simulink model "Antenna_Simulink_Block"  (R2019b)
settings: Solver=VariableStepAuto  StartTime=0.0  StopTime=0  RelTol=1e-3
undefined symbols (not defined in the file or in its folder): physconst
libraries: rfBudgetAnalyzer_lib x5, simrfV2elements x3, simrfV2util1 x3, simrfV2sources1 x1
settings Model: Creator=BLAUZON3  LastModifiedBy=BLAUZON3

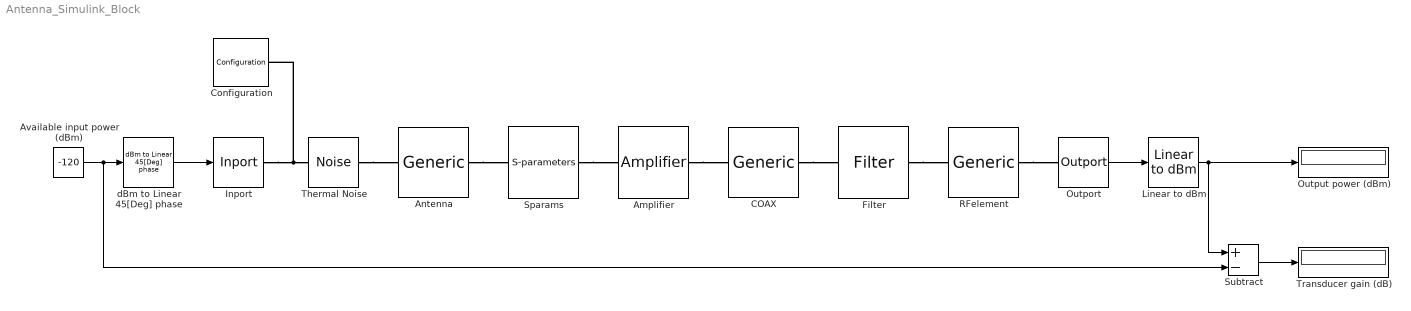
== system Antenna_Simulink_Block ==
  Amplifier : simrfV2elements/Amplifier  classname=amplifier  DataSource=Data file  File=unitygain.s2p  Paramtype=S-parameters  Sparam=[0 0;1 0]  SparamFreq=1e9 Hz  SparamZ0=50  Residues=0  Poles=0  DF={0 0; 1 0}  Source_linear_gain=Available power gain  linear_gain=12 dB  Zin=50  Zout=50  Source_Poly=Even and odd order  Poly_Coeffs=[0 1]  IPType=Output  IP2=Inf dBm  IP3=Inf dBm  P1dB=inf dBm  Psat=inf dBm  Gcomp=inf dBm  InternalGrounding=on  SourceFreq=Extracted from data source  PlotFreq=[1e9:1e6:3e9] Hz  PlotType=X-Y plane  YParam1=S11  YFormat1=Magnitude (decibels)  YParam2=None  YFormat2=Magnitude (decibels)  YOption=Linear  XOption=Linear  SparamRepresentation=Time domain (rationalfit)  FitTol=-40  FitOpt=Fit individually  AutoImpulseLength=on  ImpulseLength=1e-10 s  MagModeling=off  AddNoise=on  NoiseType=Noise figure  NoiseDist=White  NF=0  MinNF=0  Gopt=0  RN=0  CarrierFreq=0 Hz  NoiseAutoImpulseLength=on  NoiseImpulseLength=1e-10 s  SpecifyOpFreq=off  OpFreq=0 Hz
      settings: SourceProductName=RF Blockset  SourceProductBaseCode=RB
  Antenna : rfBudgetAnalyzer_lib/Generic  Gain=24  NF=0  OIP3=Inf  Zin=50  Zout=50
      settings: SourceProductName=RF Blockset  SourceProductBaseCode=RB
  Available input power (dBm) : Constant  Value=-120
  COAX : rfBudgetAnalyzer_lib/Generic  Gain=-6  NF=0  OIP3=Inf  Zin=50  Zout=50
      settings: SourceProductName=RF Blockset  SourceProductBaseCode=RB
  Configuration : simrfV2util1/Configuration  AutoFreq=on  Tones=[] Hz  Harmonics=[]  NormalizeCarrierPower=on  SolverType=Auto  UseCCode=on  StepSize=(1/20000000)/8 s  AddNoise=on  defaultRNG=on  Seed=0  Temperature=290.0 K  SolverDelFlag=0  AbsTol=1e-6  RelTol=1e-3  MaxIter=10  ErrorEstimationType=2-norm over all variables  EnableInterpFilter=on  HiddenFIRfilterControllerParam=off  SmallSignalApprox=off  AllSimFreqs=on  SimFreqs=[] Hz  SimFreqsInternal=[]  SamplesPerFrame=1
      settings: SourceProductName=RF Blockset  SourceProductBaseCode=RB
  Filter : simrfV2elements/Filter  classname=filter  DesignMethod=Butterworth  ResponseType=Bandpass  Implementation=LC Tee  ImplementationIdeal=Constant per carrier  ImplementationRational=Transfer function  UseFilterOrder=on  FilterOrder=3  PassFreq_lp=1 GHz  PassFreq_hp=2 GHz  PassFreq_bp=[5.8 6] GHz  PassFreq_bs=[1 4] GHz  PassAtten=3.0103  StopFreq_lp=2 GHz  StopFreq_hp=1 GHz  StopFreq_bp=[1.5 3.5] GHz  StopFreq_bs=[2.1 2.9] GHz  StopAtten=40  Rsrc=50  Rload=50  AutoImpulseLength=on  ImpulseLength=1e-10 s  InternalGrounding=on  PlotFuncLeft=Voltage transfer  PlotLeftForm=Magnitude (decibels)  PlotRightOnVT=None  PlotRightNoTD=None  PlotRightNoGD=None  PlotRightNoIR=None  PlotRightNoSR=None  PlotRightForm=Magnitude (decibels)  FreqPoints=logspace(0,10,101)  Freq_unit=Hz  TimePoints=linspace(0,1,1e6+1)  Time_unit=s  XaxisScale=Linear  YaxisScale=Linear
      settings: SourceProductName=RF Blockset  SourceProductBaseCode=RB
  Inport : simrfV2util1/Inport  SimulinkInputSignalType=Power  CarrierFreq=5.9 GHz  ZS=50  InternalGrounding=on
      settings: SourceProductName=RF Blockset  SourceProductBaseCode=RB
  Linear to dBm : rfBudgetAnalyzer_lib/Linear to dBm  SystemSampleTime=-1  Latency=0  AutoFrameSizeCalculation=off
      settings: SourceProductName=RF Blockset  SourceProductBaseCode=RB
  Outport : simrfV2util1/Outport  SensorType=Power  OutputFormat=Complex Baseband  CarrierFreq=5.9 GHz  ZL=50  InternalGrounding=on  StepSize=1e-6 s  AutoStep=on
      settings: SourceProductName=RF Blockset  SourceProductBaseCode=RB
  Output power (dBm) : Display
  RFelement : rfBudgetAnalyzer_lib/Generic  Gain=0  NF=0  OIP3=Inf  Zin=50  Zout=50
      settings: SourceProductName=RF Blockset  SourceProductBaseCode=RB
  Sparams : simrfV2elements/S-parameters  classname=sparam_element  DataSource=Data file  File=sparam.s2p  Paramtype=S-parameters  Sparam=[0 0;1 0]  SparamFreq=1e9 Hz  SparamZ0=50  Residues=0  Poles=0  DF={0 0; 1 0}  FitOpt=Share all poles  FitTol=-40  SourceFreq=Extracted from data source  PlotFreq=[1e9:1e6:3e9] Hz  PlotType=X-Y plane  YParam1=S11  YFormat1=Magnitude (decibels)  YParam2=None  YFormat2=Magnitude (decibels)  YOption=Linear  XOption=Linear  AddNoise=on  InternalGrounding=on  SparamRepresentation=Time domain (rationalfit)  AutoImpulseLength=on  ImpulseLength=1e-10 s  MagModeling=off
      settings: SourceProductName=RF Blockset  SourceProductBaseCode=RB
  Subtract : Sum  Inputs=+-
  Thermal Noise : simrfV2sources1/Noise  SimulinkInputSignalType=Ideal voltage  NoiseType=White  NoisePSD=4*physconst('Boltzmann')*290*50  CarrierFreq=0 Hz  AutoImpulseLength=on  ImpulseLength=1e-10 s  InternalGrounding=off
      settings: SourceProductName=RF Blockset  SourceProductBaseCode=RB
  Transducer gain (dB) : Display
  dBm to Linear 45[Deg] phase : rfBudgetAnalyzer_lib/dBm to Linear 45[Deg] phase  SystemSampleTime=-1  Latency=0  AutoFrameSizeCalculation=off
      settings: SourceProductName=RF Blockset  SourceProductBaseCode=RB
  wires:
  Available input power (dBm)/1 -> dBm to Linear 45[Deg] phase/1, Subtract/2
  dBm to Linear 45[Deg] phase/1 -> Inport/1
  Outport/1 -> Linear to dBm/1
  Linear to dBm/1 -> Output power (dBm)/1, Subtract/1
  Subtract/1 -> Transducer gain (dB)/1
  connections:
  Configuration/LConn1 -- Inport/RConn1 -- Thermal Noise/RConn1
  Thermal Noise/LConn1 -- Antenna/LConn1
  Antenna/RConn1 -- Sparams/LConn1
  Sparams/RConn1 -- Amplifier/LConn1
  Amplifier/RConn1 -- COAX/LConn1
  COAX/RConn1 -- Filter/LConn1
  Filter/RConn1 -- RFelement/LConn1
  RFelement/RConn1 -- Outport/LConn1
